simulink model "sf_multiword_fixpt"  (Simulink 7.6)
settings: Solver=FixedStepDiscrete  StartTime=0.0  StopTime=10.0  RelTol=1e-3
libraries: simulink x1
settings Model: Creator=The MathWorks Inc.
settings DebuggingCC: SolverPrmCheckMsg=none  StrictBusMsg=Warning
settings HardwareCC: ProdBitPerLong=64  ProdHWDeviceType=Generic->Custom  TargetHWDeviceType=32-bit Generic
settings SFSimCC: SimParseCustomCode=off

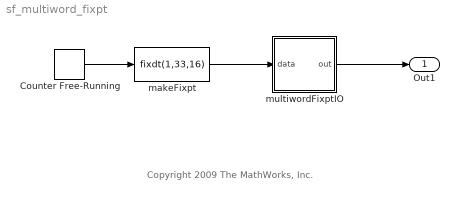
== system sf_multiword_fixpt ==
  note: Copyright 2009 The MathWorks, Inc.
  Counter Free-Running : simulink/Sources/Counter Free-Running  SystemSampleTime=-1  NumBits=16  tsamp=-1
  makeFixpt : DataTypeConversion  OutDataTypeStr=fixdt(1,33,16)
  multiwordFixptIO : Stateflow chart  TreatAsAtomicUnit=on
  Out1 : Outport
  wires:
  multiwordFixptIO/1(out) -> Out1/1
  Counter Free-Running/1 -> makeFixpt/1
  makeFixpt/1 -> multiwordFixptIO/1(data)

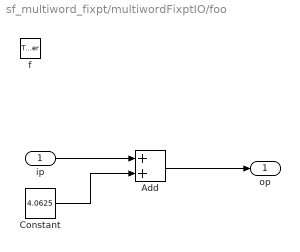
== system sf_multiword_fixpt/multiwordFixptIO/foo ==
  ip : Inport  OutDataTypeStr=fixdt(1,33,16)
  f : TriggerPort  TriggerType=function-call
      settings: CopyFcn=set_param(gcbh,'PreDeleteFcn','')  PreDeleteFcn=Stateflow.SLINSF.SimulinkMan.unsafePredeleteFcn
  Add : Sum  OutDataTypeStr=fixdt(1,33,16)
  Constant : Constant  Value=4.0625  OutDataTypeStr=fixdt(1,16,4)
  op : Outport
  wires:
  ip/1 -> Add/1
  Constant/1 -> Add/2
  Add/1 -> op/1

== stateflow chart multiwordFixptIO ==
  state A
    du:
    out = foo(data);
  state op = foo(ip) [function]
  data: ip function_input fixdt(1,33,16); op function_output double; data input fixdt(1,33,16); out output fixdt(1,33,16)
